simulink model "constant"  (R2023a)
settings: Solver=VariableStepAuto  StartTime=0.0  StopTime=10.0  RelTol=1e-3
settings Model: Creator=ian920201  LastModifiedBy=ian920201

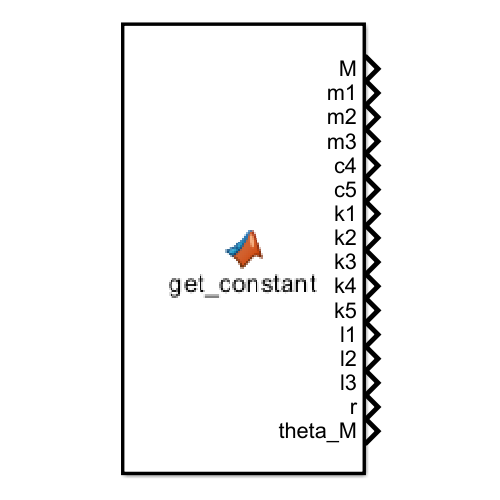
[thumbnail: Simulink's stored preview of the top-level diagram]
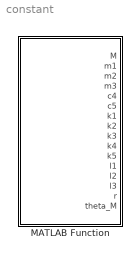
== system constant ==
  MATLAB Function : MATLAB Function  TreatAsAtomicUnit=on

== matlab function constant/MATLAB Function ==
  data: M output; m1 output; m2 output; m3 output; c4 output; c5 output; k1 output; k2 output; k3 output; k4 output; k5 output; l1 output; l2 output; l3 output; r output; theta_M output
function [M, m1, m2, m3, c4, c5, k1, k2, k3, k4, k5, l1, l2, l3, r, theta_M] = get_constant()

M = 60000;
m1 = 60;
m2 = 60;
m3 = 60;
c4 = 25000;
c5 = 25000;
k1 = 150000;
k2 = 150000;
k3 = 150000;
k4 = 150000;
k5 = 150000;
l1 = 5;
l2 = 5;
l3 = 5;
r = 100;
theta_M = deg2rad(20);
